simulink model "complete"  (R2019b)
settings: Solver=VariableStepAuto  StartTime=0.0  StopTime=200  RelTol=1e-3
values from neighbouring files (symbols this model uses):
  battery =     [battery.mat]    (also in batteryModel_Sfcn.m = block.DialogPrm(1).Data)
  controllers =     [controllers.mat]
  IC = block.DialogPrm(2).Data    [Dynamics.m]    (also in IC_HoverAt10ftOcto.mat = ; IC_HoverAt10ftOctoWithMotorControl.mat = )
  Motor =     [DJI4114_400kv_BLDC_Motor.mat]
  octomodel =     [octoModel.mat]
undefined symbols (not defined in the file or in its folder): DiscIntNeverNeededParam
libraries: simulink x1
(part 1 of 2)
settings Model: Creator=Researcher  LastModifiedBy=darrahts
settings DataIOCC: ReturnWorkspaceOutputs=off
settings DebuggingCC: ArithmeticOperatorsInVariantConditions=warning
settings SFSimCC: SimUseLocalCustomCode=off  CustomCodeUndefinedFunction=UseInterfaceOnly
settings RTWCC: RTWUseLocalCustomCode=off

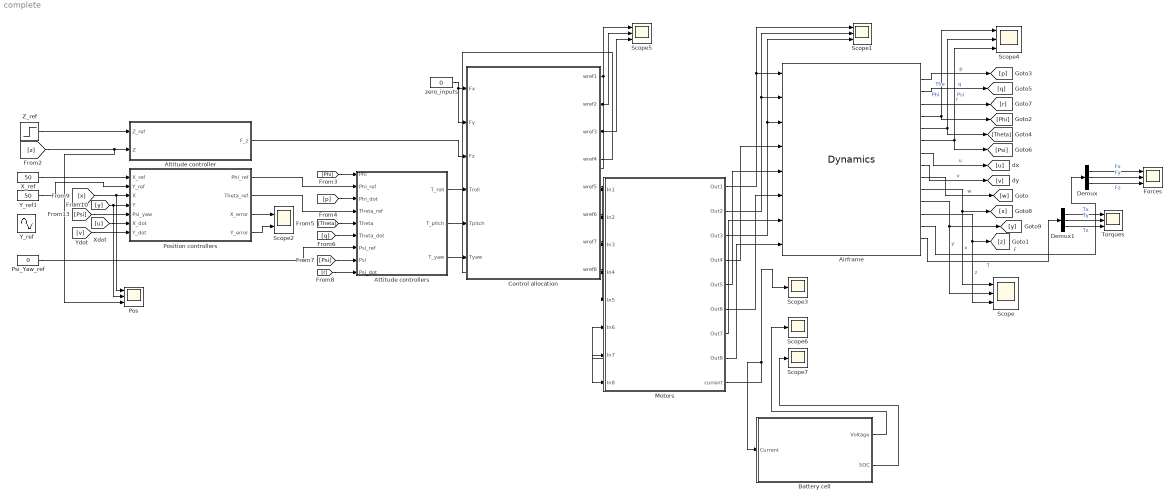
== system complete ==
  Airframe : M-S-Function  FunctionName=Dynamics  Parameters=octomodel, IC
  Altitude controller : Subsystem
  Attitude controllers : Subsystem
  Battery cell : Subsystem
  Control allocation : MATLAB Function  TreatAsAtomicUnit=on
  Demux : Demux  Outputs=3
  Demux1 : Demux  Outputs=3
  Forces : Scope  NumInputPorts=3
  Motors : Subsystem
  Pos : Scope  NumInputPorts=3
  Position controllers : Subsystem
  Psi_Yaw_ref : Constant  Value=0
  Scope{,1,4..5} (4 alike) : Scope  NumInputPorts=3
  Scope2 : Scope  NumInputPorts=2
  Scope3 : Scope
  Scope6 : Scope
  Scope7 : Scope
  Torques : Scope  NumInputPorts=3
  X_ref : Constant  Value=50
  Y_ref : Sin  Amplitude=2  Frequency=0.1  SampleTime=0
  Y_ref1 : Constant  Value=50
  Z_ref : Step  Before=3  After=3  SampleTime=0
  zero_inputs : Constant  Value=0
  wires:
  Airframe/1 -> [p]  "p"
  Airframe/2 -> [q]  "q"
  Airframe/3 -> [r]  "r"
  Airframe/4 -> [Phi], Scope4/1  "Phi"
  Airframe/5 -> [Theta], Scope4/2  "The"
  Airframe/6 -> [Psi], Scope4/3  "Psi"
  Airframe/11 -> [y], Scope/2  "y"
  Airframe/12 -> [z], Scope/3  "z"
  Airframe/7 -> [u]  "u"
  Airframe/10 -> [x], Scope/1  "x"
  Airframe/9 -> [w]  "w"
  Airframe/8 -> [v]  "v"
  Motors/3(Out3) -> Scope1/3, Airframe/3
  Control allocation/1(wref1) -> Scope5/1, Motors/1(In1)
  Control allocation/2(wref2) -> Scope5/2, Motors/2(In2)
  Motors/1(Out1) -> Scope1/1, Airframe/1
  Control allocation/3(wref3) -> Scope5/3, Motors/3(In3)
  Control allocation/4(wref4) -> Motors/4(In4)
  Control allocation/5(wref5) -> Motors/5(In5)
  Control allocation/6(wref6) -> Motors/6(In6)
  Control allocation/7(wref7) -> Motors/7(In7)
  Control allocation/8(wref8) -> Motors/8(In8)
  Motors/8(Out8) -> Airframe/8
  Motors/7(Out7) -> Airframe/7
  Motors/6(Out6) -> Airframe/6
  Motors/5(Out5) -> Airframe/5
  Motors/4(Out4) -> Airframe/4
  Motors/2(Out2) -> Scope1/2, Airframe/2
  zero_inputs/1 -> Control allocation/2(Fy), Control allocation/1(Fx)
  [y] -> Position controllers/4(Y), Pos/2
  Y_ref1/1 -> Position controllers/2(Y_ref)
  X_ref/1 -> Position controllers/1(X_ref)
  [x] -> Pos/1, Position controllers/3(X)
  [Psi] -> Position controllers/5(Psi_yaw)
  [v] -> Position controllers/7(Y_dot)
  [u] -> Position controllers/6(X_dot)
  Position controllers/3(X_error) -> Scope2/1
  Position controllers/4(Y_error) -> Scope2/2
  Z_ref/1 -> Altitude controller/1(Z_ref)
  [z] -> Pos/3, Altitude controller/2(Z)
  Altitude controller/1(F_z) -> Control allocation/3(Fz)
  [Phi] -> Attitude controllers/1(Phi)
  Position controllers/1(Phi_ref) -> Attitude controllers/2(Phi_ref)
  [p] -> Attitude controllers/3(Phi_dot)
  Position controllers/2(Theta_ref) -> Attitude controllers/4(Theta_ref)
  [Theta] -> Attitude controllers/5(Theta)
  [q] -> Attitude controllers/6(Theta_dot)
  Psi_Yaw_ref/1 -> Attitude controllers/7(Psi_ref)
  [Psi] -> Attitude controllers/8(Psi)
  [r] -> Attitude controllers/9(Psi_dot)
  Attitude controllers/1(T_roll) -> Control allocation/4(Troll)
  Attitude controllers/2(T_pitch) -> Control allocation/5(Tpitch)
  Attitude controllers/3(T_yaw) -> Control allocation/6(Tyaw)
  Motors/9(current) -> Scope3/1, Battery cell/1(Current)
  Battery cell/1(Voltage) -> Scope6/1
  Battery cell/2(SOC) -> Scope7/1
  Airframe/13 -> Demux/1  "F"
  Airframe/14 -> Demux1/1  "T"
  Demux/1 -> Forces/1  "Fx"
  Demux/2 -> Forces/2  "Fy"
  Demux/3 -> Forces/3  "Fz"
  Demux1/1 -> Torques/1  "Tx"
  Demux1/2 -> Torques/2  "Ty"
  Demux1/3 -> Torques/3  "Tz"

== system complete/Altitude controller ==
  Z_ref : Inport
  Z : Inport  Port=2
  Add : Sum
  Add2 : Sum  Inputs=+-
  Constant2 : Constant  Value=octomodel.g*octomodel.mass
  PID Controller : simulink/Continuous/PID Controller  Controller=PID  Form=Parallel  TimeDomain=Discrete-time  SampleTime=0.01  IntegratorMethod=Forward Euler  FilterMethod=Forward Euler  ControllerParametersSource=internal  P=controllers.altitude.kp  I=controllers.altitude.ki  D=controllers.altitude.kd  UseFilter=on  N=100  TunerSelectOption=Transfer Function Based (PID Tuner App)  InitialConditionSource=internal  InitialConditionForIntegrator=0  InitialConditionForFilter=0  DifferentiatorICPrevScaledInput=0  ExternalReset=none  TrackingMode=off  Kt=1  LimitOutput=off  UpperSaturationLimit=inf  LowerSaturationLimit=0  LinearizeAsGain=on  AntiWindupMode=none  Kb=1  POutMin=[]  POutMax=[]  IOutMin=[]  IOutMax=[]  DOutMin=[]  DOutMax=[]  NOutMin=[]  NOutMax=[]  SumOutMin=[]  SumOutMax=[]  SaturationOutMin=[]  SaturationOutMax=[]  PParamMin=[]  PParamMax=[]  IParamMin=[]  IParamMax=[]  DParamMin=[]  DParamMax=[]  NParamMin=[]  NParamMax=[]  KbParamMin=[]  KbParamMax=[]  KtParamMin=[]  KtParamMax=[]  KbOutMin=[]  KbOutMax=[]  KtOutMin=[]  KtOutMax=[]  IntegratorOutMin=[]  IntegratorOutMax=[]  FilterOutMin=[]  FilterOutMax=[]  SumI1OutMin=[]  SumI1OutMax=[]  SumI2OutMin=[]  SumI2OutMax=[]  SumI3OutMin=[]  SumI3OutMax=[]  SumI4OutMin=[]  SumI4OutMax=[]  SumDOutMin=[]  SumDOutMax=[]  DifferentiatorOutMin=[]  DifferentiatorOutMax=[]  FilterDiffOutCoefMin=[]  FilterDiffOutCoefMax=[]  ReciprocalOutMin=[]  ReciprocalOutMax=[]  SumDenOutMin=[]  SumDenOutMax=[]  SumNumOutMin=[]  SumNumOutMax=[]  DivideOutMin=[]  DivideOutMax=[]  IntegratorContinuousStateAttributes=''  IntegratorStateMustResolveToSignalObject=off  IntegratorRTWStateStorageClass=Auto  FilterContinuousStateAttributes=''  FilterStateMustResolveToSignalObject=off  FilterRTWStateStorageClass=Auto  ParallelPVariant=InternalParameters  IdealPVariant=Disabled  IVariant=InternalParameters  DVariant=InternalParameters  IntegratorVariant=Discrete  SatVariant=Disabled  AWVariant=Passthrough  PCopyVariant=Disabled  TRVariant=Disabled  FdbkBlocksVariant=Forward  IdealPFdbkVariant=Disabled  SatFdbkVariant=Disabled  DerivativeFilterVariant=ForwardEulerFilter  NVariant=InternalParameters  NCopyVariant=Disabled  FilterICVariant=InternalICsFilter  IntegratorICVariant=InternalICs  ExternalResetVariant=Disabled  TRSumVariant=Passthrough  SumFdbkVariant=Disabled  SumVariant=Sum_PID
  F_z : Outport  VectorParamsAs1DForOutWhenUnconnected=off
  wires:
  Add2/1 -> PID Controller/1
  Constant2/1 -> Add/1
  Z/1 -> Add2/2
  Add/1 -> F_z/1
  Z_ref/1 -> Add2/1
  PID Controller/1 -> Add/2

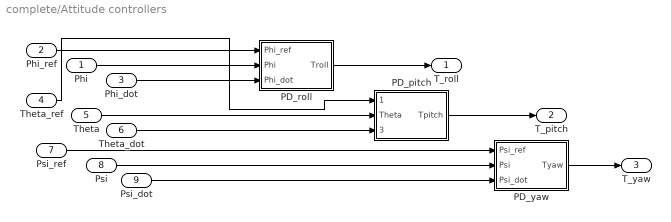
== system complete/Attitude controllers ==
  Phi : Inport
  Phi_ref : Inport  Port=2
  Phi_dot : Inport  Port=3
  Theta_ref : Inport  Port=4
  Theta : Inport  Port=5
  Theta_dot : Inport  Port=6
  Psi_ref : Inport  Port=7
  Psi : Inport  Port=8
  Psi_dot : Inport  Port=9
  PD_pitch : Subsystem
  PD_roll : Subsystem
  PD_yaw : Subsystem
  T_roll : Outport  VectorParamsAs1DForOutWhenUnconnected=off
  T_pitch : Outport  Port=2  VectorParamsAs1DForOutWhenUnconnected=off
  T_yaw : Outport  Port=3  VectorParamsAs1DForOutWhenUnconnected=off
  wires:
  PD_yaw/1(Tyaw) -> T_yaw/1
  PD_roll/1(Troll) -> T_roll/1
  Theta_ref/1 -> PD_pitch/1(Theta_ref)
  Theta_dot/1 -> PD_pitch/3(Theta_dot)
  PD_pitch/1(Tpitch) -> T_pitch/1
  Phi/1 -> PD_roll/2(Phi)
  Psi_dot/1 -> PD_yaw/3(Psi_dot)
  Psi_ref/1 -> PD_yaw/1(Psi_ref)
  Theta/1 -> PD_pitch/2(Theta)
  Phi_dot/1 -> PD_roll/3(Phi_dot)
  Psi/1 -> PD_yaw/2(Psi)
  Phi_ref/1 -> PD_roll/1(Phi_ref)

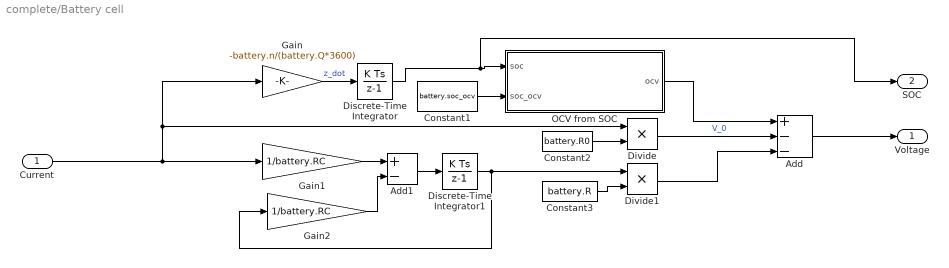
== system complete/Battery cell ==
  Current : Inport
  Add : Sum  Inputs=+--
  Add1 : Sum  Inputs=+-
  Constant1 : Constant  Value=battery.soc_ocv
  Constant2 : Constant  Value=battery.R0
  Constant3 : Constant  Value=battery.R
  Discrete-Time Integrator : DiscreteIntegrator  InitialCondition=1  ICPrevOutput=DiscIntNeverNeededParam  ICPrevScaledInput=DiscIntNeverNeededParam
  Discrete-Time Integrator1 : DiscreteIntegrator  ICPrevOutput=DiscIntNeverNeededParam  ICPrevScaledInput=DiscIntNeverNeededParam
  Divide : Product  Inputs=**
  Divide1 : Product  Inputs=**
  Gain : Gain  Gain=-battery.n/(battery.Q*3600)
  Gain1 : Gain  Gain=1/battery.RC
  Gain2 : Gain  Gain=1/battery.RC
  OCV from SOC : MATLAB Function  TreatAsAtomicUnit=on
  Voltage : Outport  VectorParamsAs1DForOutWhenUnconnected=off
  SOC : Outport  Port=2  VectorParamsAs1DForOutWhenUnconnected=off
  wires:
  Constant2/1 -> Divide/2
  Constant1/1 -> OCV from SOC/2(soc_ocv)
  Divide/1 -> Add/2  "V_0"
  OCV from SOC/1(ocv) -> Add/1
  Add1/1 -> Discrete-Time Integrator1/1
  Gain1/1 -> Add1/1
  Constant3/1 -> Divide1/2
  Divide1/1 -> Add/3
  Gain2/1 -> Add1/2
  Discrete-Time Integrator/1 -> SOC/1, OCV from SOC/1(soc)
  Gain/1 -> Discrete-Time Integrator/1  "z_dot"
  Discrete-Time Integrator1/1 -> Gain2/1, Divide1/1
  Add/1 -> Voltage/1
  Current/1 -> Gain1/1, Gain/1, Divide/1

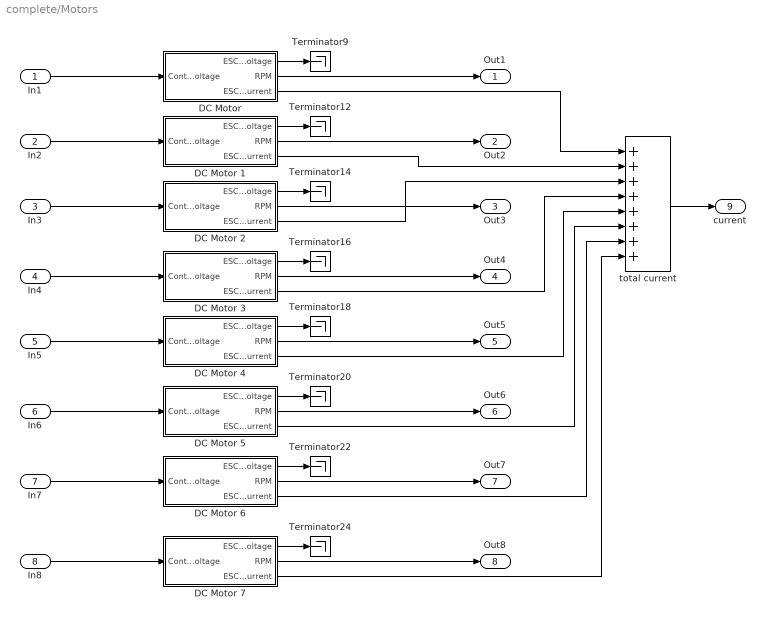
== system complete/Motors ==
  In1 : Inport
  In2 : Inport  Port=2
  In3 : Inport  Port=3
  In4 : Inport  Port=4
  In5 : Inport  Port=5
  In6 : Inport  Port=6
  In7 : Inport  Port=7
  In8 : Inport  Port=8
  "DC Motor " : Subsystem
  DC Motor 1 : Subsystem
  DC Motor 2 : Subsystem
  DC Motor 3 : Subsystem
  DC Motor 4 : Subsystem
  DC Motor 5 : Subsystem
  DC Motor 6 : Subsystem
  DC Motor 7 : Subsystem
  Terminator{9,12,14,16,18,20,22,24} (8 alike) : Terminator
  total current : Sum  Inputs=++++++++
  Out1 : Outport  VectorParamsAs1DForOutWhenUnconnected=off
  Out2 : Outport  Port=2  VectorParamsAs1DForOutWhenUnconnected=off
  Out3 : Outport  Port=3  VectorParamsAs1DForOutWhenUnconnected=off
  Out4 : Outport  Port=4  VectorParamsAs1DForOutWhenUnconnected=off
  Out5 : Outport  Port=5  VectorParamsAs1DForOutWhenUnconnected=off
  Out6 : Outport  Port=6  VectorParamsAs1DForOutWhenUnconnected=off
  Out7 : Outport  Port=7  VectorParamsAs1DForOutWhenUnconnected=off
  Out8 : Outport  Port=8  VectorParamsAs1DForOutWhenUnconnected=off
  current : Outport  Port=9  VectorParamsAs1DForOutWhenUnconnected=off
  wires:
  DC Motor 4/1(ESC Voltage) -> Terminator18/1
  DC Motor 5/3(ESC Current) -> total current/6
  DC Motor 6/3(ESC Current) -> total current/7
  DC Motor 6/1(ESC Voltage) -> Terminator22/1
  DC Motor 5/1(ESC Voltage) -> Terminator20/1
  DC Motor 4/3(ESC Current) -> total current/5
  DC Motor 7/3(ESC Current) -> total current/8
  "DC Motor "/3(ESC Current) -> total current/1
  "DC Motor "/1(ESC Voltage) -> Terminator9/1
  DC Motor 1/3(ESC Current) -> total current/2
  DC Motor 1/1(ESC Voltage) -> Terminator12/1
  DC Motor 2/1(ESC Voltage) -> Terminator14/1
  DC Motor 3/3(ESC Current) -> total current/4
  DC Motor 2/3(ESC Current) -> total current/3
  DC Motor 4/2(RPM) -> Out5/1
  DC Motor 3/1(ESC Voltage) -> Terminator16/1
  DC Motor 7/1(ESC Voltage) -> Terminator24/1
  DC Motor 6/2(RPM) -> Out7/1
  DC Motor 1/2(RPM) -> Out2/1
  DC Motor 2/2(RPM) -> Out3/1
  DC Motor 3/2(RPM) -> Out4/1
  DC Motor 5/2(RPM) -> Out6/1
  DC Motor 7/2(RPM) -> Out8/1
  "DC Motor "/2(RPM) -> Out1/1
  In1/1 -> "DC Motor "/1(Control  Voltage)
  In7/1 -> DC Motor 6/1(Control  Voltage)
  In8/1 -> DC Motor 7/1(Control  Voltage)
  In6/1 -> DC Motor 5/1(Control  Voltage)
  In5/1 -> DC Motor 4/1(Control  Voltage)
  In4/1 -> DC Motor 3/1(Control  Voltage)
  In3/1 -> DC Motor 2/1(Control  Voltage)
  In2/1 -> DC Motor 1/1(Control Voltage)
  total current/1 -> current/1

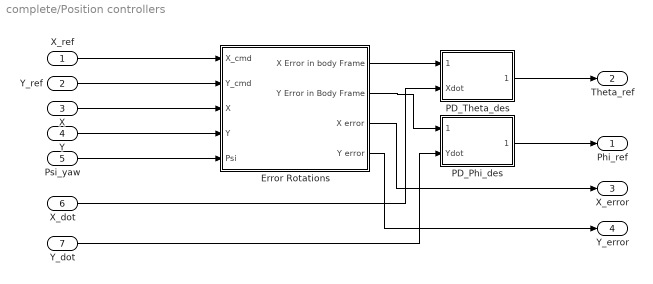
== system complete/Position controllers ==
  X_ref : Inport
  Y_ref : Inport  Port=2
  X : Inport  Port=3
  Y : Inport  Port=4
  Psi_yaw : Inport  Port=5
  X_dot : Inport  Port=6
  Y_dot : Inport  Port=7
  Error Rotations : Subsystem
  PD_Phi_des : Subsystem
  PD_Theta_des : Subsystem
  Phi_ref : Outport  VectorParamsAs1DForOutWhenUnconnected=off
  Theta_ref : Outport  Port=2  VectorParamsAs1DForOutWhenUnconnected=off
  X_error : Outport  Port=3  VectorParamsAs1DForOutWhenUnconnected=off
  Y_error : Outport  Port=4  VectorParamsAs1DForOutWhenUnconnected=off
  wires:
  Y/1 -> Error Rotations/4(Y)
  Y_ref/1 -> Error Rotations/2(Y_cmd)
  Error Rotations/4("Y error ") -> Y_error/1
  Error Rotations/3(X error) -> X_error/1
  Error Rotations/1(X Error in body Frame) -> PD_Theta_des/1(Xdot_ref)
  X/1 -> Error Rotations/3(X)
  Y_dot/1 -> PD_Phi_des/2(Ydot)
  PD_Phi_des/1(Phi_des) -> Phi_ref/1
  Error Rotations/2(Y Error in Body Frame) -> PD_Phi_des/1(Ydot_ref)
  Psi_yaw/1 -> Error Rotations/5(Psi)
  PD_Theta_des/1(Theta_des) -> Theta_ref/1
  X_dot/1 -> PD_Theta_des/2(Xdot)
  X_ref/1 -> Error Rotations/1(X_cmd)

== system complete/Attitude controllers/PD_pitch ==
  Theta_ref : Inport
  Theta : Inport  Port=2
  Theta_dot : Inport  Port=3
  Add : Sum  Inputs=-+
  Gain : Gain  Gain=controllers.attitude.pitch.kp
  Gain1 : Gain  Gain=controllers.attitude.pitch.kp
  Gain2 : Gain  Gain=-1
  Sum : Sum  Inputs=|++
  Tpitch : Outport  VectorParamsAs1DForOutWhenUnconnected=off
  wires:
  Gain2/1 -> Tpitch/1
  Gain/1 -> Sum/1
  Theta/1 -> Add/2
  Add/1 -> Gain/1
  Gain1/1 -> Sum/2
  Sum/1 -> Gain2/1
  Theta_dot/1 -> Gain1/1
  Theta_ref/1 -> Add/1

== system complete/Attitude controllers/PD_roll ==
  Phi_ref : Inport
  Phi : Inport  Port=2
  Phi_dot : Inport  Port=3
  Add : Sum  Inputs=-+
  Gain : Gain  Gain=controllers.attitude.roll.kp
  Gain1 : Gain  Gain=controllers.attitude.roll.kd
  Gain2 : Gain  Gain=-1
  Sum : Sum  Inputs=|++
  Troll : Outport  VectorParamsAs1DForOutWhenUnconnected=off
  wires:
  Phi_ref/1 -> Add/1
  Phi_dot/1 -> Gain1/1
  Sum/1 -> Gain2/1
  Gain1/1 -> Sum/2
  Add/1 -> Gain/1
  Phi/1 -> Add/2
  Gain/1 -> Sum/1
  Gain2/1 -> Troll/1

== system complete/Attitude controllers/PD_yaw ==
  Psi_ref : Inport
  Psi : Inport  Port=2
  Psi_dot : Inport  Port=3
  Add : Sum  Inputs=-+
  Gain : Gain  Gain=controllers.attitude.yaw.kp
  Gain1 : Gain  Gain=controllers.attitude.yaw.kp
  Gain2 : Gain  Gain=-1
  Sum : Sum  Inputs=|++
  Tyaw : Outport  VectorParamsAs1DForOutWhenUnconnected=off
  wires:
  Psi_ref/1 -> Add/1
  Psi_dot/1 -> Gain1/1
  Sum/1 -> Gain2/1
  Gain1/1 -> Sum/2
  Add/1 -> Gain/1
  Psi/1 -> Add/2
  Gain/1 -> Sum/1
  Gain2/1 -> Tyaw/1

== system complete/Motors/DC Motor  ==
  Control  Voltage : Inport
  Convert rad/s to rmp : Gain  Gain=60/(2*pi)
  Electrical part : Subsystem
  Mechanical part : Subsystem
  Scope : Scope
  Scope3 : Scope
  Scope7 : Scope  NumInputPorts=3
  StaticTfric : Constant  Value=0
  ESC Voltage : Outport  VectorParamsAs1DForOutWhenUnconnected=off
  RPM : Outport  Port=2  VectorParamsAs1DForOutWhenUnconnected=off
  ESC Current : Outport  Port=3  VectorParamsAs1DForOutWhenUnconnected=off
  wires:
  StaticTfric/1 -> Mechanical part/1(Static Friction Torque)
  Convert rad/s to rmp/1 -> RPM/1
  Electrical part/1(Electrical Torque) -> Scope3/1, Mechanical part/2(Electrical Torque)
  Mechanical part/1(w angular speed) -> Electrical part/2(w angular speed), Scope7/1, Convert rad/s to rmp/1
  Mechanical part/3(Torque) -> Scope7/3
  Mechanical part/2(Thrust) -> Scope/1, Scope7/2
  Electrical part/2(current) -> ESC Current/1
  Control  Voltage/1 -> ESC Voltage/1, Electrical part/1(ESC voltage)

== system complete/Motors/DC Motor 1 ==
  Control Voltage : Inport
  Convert rad/s to rmp : Gain  Gain=60/(2*pi)
  Electrical part : Subsystem
  Mechanical part : Subsystem
  Scope : Scope
  Scope3 : Scope
  Scope7 : Scope  NumInputPorts=3
  StaticTfric : Constant  Value=0
  ESC Voltage : Outport  VectorParamsAs1DForOutWhenUnconnected=off
  RPM : Outport  Port=2  VectorParamsAs1DForOutWhenUnconnected=off
  ESC Current : Outport  Port=3  VectorParamsAs1DForOutWhenUnconnected=off
  wires:
  Control Voltage/1 -> Electrical part/1(ESC voltage), ESC Voltage/1
  Electrical part/2(current) -> ESC Current/1
  Mechanical part/2(Thrust) -> Scope7/2, Scope/1
  Mechanical part/3(Torque) -> Scope7/3
  Mechanical part/1(w angular speed) -> Convert rad/s to rmp/1, Scope7/1, Electrical part/2(w angular speed)
  Electrical part/1(Electrical Torque) -> Mechanical part/2(Electrical Torque), Scope3/1
  Convert rad/s to rmp/1 -> RPM/1
  StaticTfric/1 -> Mechanical part/1(Static Friction Torque)

== system complete/Motors/DC Motor 2 ==
  Control  Voltage : Inport
  Convert rad/s to rmp : Gain  Gain=60/(2*pi)
  Electrical part : Subsystem
  Mechanical part : Subsystem
  Scope : Scope
  Scope3 : Scope
  Scope7 : Scope  NumInputPorts=3
  StaticTfric : Constant  Value=0
  ESC Voltage : Outport  VectorParamsAs1DForOutWhenUnconnected=off
  RPM : Outport  Port=2  VectorParamsAs1DForOutWhenUnconnected=off
  ESC Current : Outport  Port=3  VectorParamsAs1DForOutWhenUnconnected=off
  wires:
  StaticTfric/1 -> Mechanical part/1(Static Friction Torque)
  Convert rad/s to rmp/1 -> RPM/1
  Electrical part/1(Electrical Torque) -> Scope3/1, Mechanical part/2(Electrical Torque)
  Mechanical part/1(w angular speed) -> Electrical part/2(w angular speed), Scope7/1, Convert rad/s to rmp/1
  Mechanical part/3(Torque) -> Scope7/3
  Mechanical part/2(Thrust) -> Scope/1, Scope7/2
  Electrical part/2(current) -> ESC Current/1
  Control  Voltage/1 -> ESC Voltage/1, Electrical part/1(ESC voltage)

== system complete/Motors/DC Motor 3 ==
  Control  Voltage : Inport
  Convert rad/s to rmp : Gain  Gain=60/(2*pi)
  Electrical part : Subsystem
  Mechanical part : Subsystem
  Scope : Scope
  Scope3 : Scope
  Scope7 : Scope  NumInputPorts=3
  StaticTfric : Constant  Value=0
  ESC Voltage : Outport  VectorParamsAs1DForOutWhenUnconnected=off
  RPM : Outport  Port=2  VectorParamsAs1DForOutWhenUnconnected=off
  ESC Current : Outport  Port=3  VectorParamsAs1DForOutWhenUnconnected=off
  wires:
  Control  Voltage/1 -> Electrical part/1(ESC voltage), ESC Voltage/1
  Electrical part/2(current) -> ESC Current/1
  Mechanical part/2(Thrust) -> Scope7/2, Scope/1
  Mechanical part/3(Torque) -> Scope7/3
  Mechanical part/1(w angular speed) -> Convert rad/s to rmp/1, Scope7/1, Electrical part/2(w angular speed)
  Electrical part/1(Electrical Torque) -> Mechanical part/2(Electrical Torque), Scope3/1
  Convert rad/s to rmp/1 -> RPM/1
  StaticTfric/1 -> Mechanical part/1(Static Friction Torque)

== system complete/Motors/DC Motor 4 ==
  Control  Voltage : Inport
  Convert rad/s to rmp : Gain  Gain=60/(2*pi)
  Electrical part : Subsystem
  Mechanical part : Subsystem
  Scope : Scope
  Scope3 : Scope
  Scope7 : Scope  NumInputPorts=3
  StaticTfric : Constant  Value=0
  ESC Voltage : Outport  VectorParamsAs1DForOutWhenUnconnected=off
  RPM : Outport  Port=2  VectorParamsAs1DForOutWhenUnconnected=off
  ESC Current : Outport  Port=3  VectorParamsAs1DForOutWhenUnconnected=off
  wires:
  StaticTfric/1 -> Mechanical part/1(Static Friction Torque)
  Convert rad/s to rmp/1 -> RPM/1
  Electrical part/1(Electrical Torque) -> Scope3/1, Mechanical part/2(Electrical Torque)
  Mechanical part/1(w angular speed) -> Electrical part/2(w angular speed), Scope7/1, Convert rad/s to rmp/1
  Mechanical part/3(Torque) -> Scope7/3
  Mechanical part/2(Thrust) -> Scope/1, Scope7/2
  Electrical part/2(current) -> ESC Current/1
  Control  Voltage/1 -> ESC Voltage/1, Electrical part/1(ESC voltage)

== system complete/Motors/DC Motor 5 ==
  Control  Voltage : Inport
  Convert rad/s to rmp : Gain  Gain=60/(2*pi)
  Electrical part : Subsystem
  Mechanical part : Subsystem
  Scope : Scope
  Scope3 : Scope
  Scope7 : Scope  NumInputPorts=3
  StaticTfric : Constant  Value=0
  ESC Voltage : Outport  VectorParamsAs1DForOutWhenUnconnected=off
  RPM : Outport  Port=2  VectorParamsAs1DForOutWhenUnconnected=off
  ESC Current : Outport  Port=3  VectorParamsAs1DForOutWhenUnconnected=off
  wires:
  Control  Voltage/1 -> Electrical part/1(ESC voltage), ESC Voltage/1
  Electrical part/2(current) -> ESC Current/1
  Mechanical part/2(Thrust) -> Scope7/2, Scope/1
  Mechanical part/3(Torque) -> Scope7/3
  Mechanical part/1(w angular speed) -> Convert rad/s to rmp/1, Scope7/1, Electrical part/2(w angular speed)
  Electrical part/1(Electrical Torque) -> Mechanical part/2(Electrical Torque), Scope3/1
  Convert rad/s to rmp/1 -> RPM/1
  StaticTfric/1 -> Mechanical part/1(Static Friction Torque)

== system complete/Motors/DC Motor 6 ==
  Control  Voltage : Inport
  Convert rad/s to rmp : Gain  Gain=60/(2*pi)
  Electrical part : Subsystem
  Mechanical part : Subsystem
  Scope : Scope
  Scope3 : Scope
  Scope7 : Scope  NumInputPorts=3
  StaticTfric : Constant  Value=0
  ESC Voltage : Outport  VectorParamsAs1DForOutWhenUnconnected=off
  RPM : Outport  Port=2  VectorParamsAs1DForOutWhenUnconnected=off
  ESC Current : Outport  Port=3  VectorParamsAs1DForOutWhenUnconnected=off
  wires:
  StaticTfric/1 -> Mechanical part/1(Static Friction Torque)
  Convert rad/s to rmp/1 -> RPM/1
  Electrical part/1(Electrical Torque) -> Scope3/1, Mechanical part/2(Electrical Torque)
  Mechanical part/1(w angular speed) -> Electrical part/2(w angular speed), Scope7/1, Convert rad/s to rmp/1
  Mechanical part/3(Torque) -> Scope7/3
  Mechanical part/2(Thrust) -> Scope/1, Scope7/2
  Electrical part/2(current) -> ESC Current/1
  Control  Voltage/1 -> ESC Voltage/1, Electrical part/1(ESC voltage)

== system complete/Motors/DC Motor 7 ==
  Control  Voltage : Inport
  Convert rad/s to rmp : Gain  Gain=60/(2*pi)
  Electrical part : Subsystem
  Mechanical part : Subsystem
  Scope : Scope
  Scope3 : Scope
  Scope7 : Scope  NumInputPorts=3
  StaticTfric : Constant  Value=0
  ESC Voltage : Outport  VectorParamsAs1DForOutWhenUnconnected=off
  RPM : Outport  Port=2  VectorParamsAs1DForOutWhenUnconnected=off
  ESC Current : Outport  Port=3  VectorParamsAs1DForOutWhenUnconnected=off
  wires:
  Control  Voltage/1 -> Electrical part/1(ESC voltage), ESC Voltage/1
  Electrical part/2(current) -> ESC Current/1
  Mechanical part/2(Thrust) -> Scope7/2, Scope/1
  Mechanical part/3(Torque) -> Scope7/3
  Mechanical part/1(w angular speed) -> Convert rad/s to rmp/1, Scope7/1, Electrical part/2(w angular speed)
  Electrical part/1(Electrical Torque) -> Mechanical part/2(Electrical Torque), Scope3/1
  Convert rad/s to rmp/1 -> RPM/1
  StaticTfric/1 -> Mechanical part/1(Static Friction Torque)

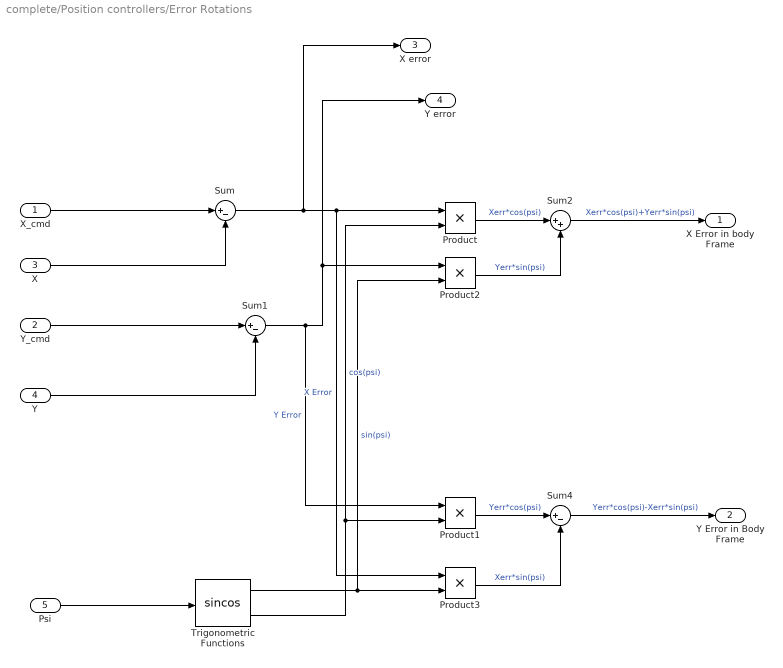
== system complete/Position controllers/Error Rotations ==
  X_cmd : Inport
  Y_cmd : Inport  Port=2
  X : Inport  Port=3
  Y : Inport  Port=4
  Psi : Inport  Port=5
  Product{,1..3} (4 alike) : Product
  Sum : Sum  Inputs=|+-
  Sum1 : Sum  Inputs=|+-
  Sum2 : Sum  Inputs=|++
  Sum4 : Sum  Inputs=|+-
  Trigonometric Functions : Trigonometry  Operator=sincos
  X Error in body Frame : Outport  VectorParamsAs1DForOutWhenUnconnected=off
  Y Error in Body Frame : Outport  Port=2  VectorParamsAs1DForOutWhenUnconnected=off
  X error : Outport  Port=3  VectorParamsAs1DForOutWhenUnconnected=off
  "Y error " : Outport  Port=4  VectorParamsAs1DForOutWhenUnconnected=off
  wires:
  Sum4/1 -> Y Error in Body Frame/1  "Yerr*cos(psi)-Xerr*sin(psi)"
  Product3/1 -> Sum4/2  "Xerr*sin(psi)"
  Sum1/1 -> "Y error "/1, Product2/1, Product1/1  "Y Error"
  Trigonometric Functions/1 -> Product2/2, Product3/2  "sin(psi)"
  Sum2/1 -> X Error in body Frame/1  "Xerr*cos(psi)+Yerr*sin(psi)"
  Y_cmd/1 -> Sum1/1
  X_cmd/1 -> Sum/1
  X/1 -> Sum/2
  Y/1 -> Sum1/2
  Sum/1 -> X error/1, Product3/1, Product/1  "X Error"
  Trigonometric Functions/2 -> Product/2, Product1/2  "cos(psi)"
  Product/1 -> Sum2/1  "Xerr*cos(psi)"
  Product2/1 -> Sum2/2  "Yerr*sin(psi)"
  Product1/1 -> Sum4/1  "Yerr*cos(psi)"
  Psi/1 -> Trigonometric Functions/1

== system complete/Position controllers/PD_Phi_des ==
  Ydot_ref : Inport
  Ydot : Inport  Port=2
  Add : Sum  Inputs=+-
  Gain : Gain
  Gain1 : Gain  Gain=.5
  Gain2 : Gain  Gain=-1
  Saturation in radians : Saturate  UpperLimit=12*pi/180  LowerLimit=-12*pi/180
  Sum : Sum  Inputs=|+-
  Phi_des : Outport  VectorParamsAs1DForOutWhenUnconnected=off
  wires:
  Saturation in radians/1 -> Phi_des/1
  Ydot_ref/1 -> Add/1
  Ydot/1 -> Add/2, Gain1/1
  Gain1/1 -> Sum/2
  Add/1 -> Gain/1
  Gain/1 -> Sum/1
  Sum/1 -> Gain2/1
  Gain2/1 -> Saturation in radians/1

== system complete/Position controllers/PD_Theta_des ==
  Xdot_ref : Inport
  Xdot : Inport  Port=2
  Add : Sum  Inputs=+-
  Gain : Gain
  Gain1 : Gain  Gain=.5
  Saturation in radians : Saturate  UpperLimit=12*pi/180  LowerLimit=-12*pi/180
  Sum : Sum  Inputs=|+-
  Theta_des : Outport  VectorParamsAs1DForOutWhenUnconnected=off
  wires:
  Sum/1 -> Saturation in radians/1
  Gain/1 -> Sum/1
  Add/1 -> Gain/1
  Gain1/1 -> Sum/2
  Xdot/1 -> Gain1/1, Add/2
  Xdot_ref/1 -> Add/1
  Saturation in radians/1 -> Theta_des/1

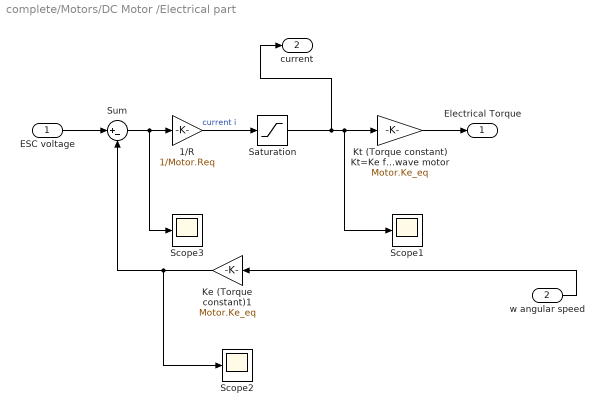
== system complete/Motors/DC Motor /Electrical part ==
  ESC voltage : Inport
  w angular speed : Inport  Port=2
  1/R : Gain  Gain=1/Motor.Req
  Ke (Torque constant)1 : Gain  Gain=Motor.Ke_eq
  Kt (Torque constant) Kt=Ke for an ideal square wave motor : Gain  Gain=Motor.Ke_eq
  Saturation : Saturate  UpperLimit=22  LowerLimit=0
  Scope1 : Scope
  Scope2 : Scope
  Scope3 : Scope
  Sum : Sum  Inputs=|+-
  Electrical Torque : Outport  VectorParamsAs1DForOutWhenUnconnected=off
  current : Outport  Port=2  VectorParamsAs1DForOutWhenUnconnected=off
  wires:
  1/R/1 -> Saturation/1  "current i"
  Sum/1 -> Scope3/1, 1/R/1
  Kt (Torque constant) Kt=Ke for an ideal square wave motor/1 -> Electrical Torque/1
  Ke (Torque constant)1/1 -> Scope2/1, Sum/2
  ESC voltage/1 -> Sum/1
  w angular speed/1 -> Ke (Torque constant)1/1
  Saturation/1 -> Scope1/1, Kt (Torque constant) Kt=Ke for an ideal square wave motor/1, current/1

== system complete/Motors/DC Motor /Mechanical part ==
  Static Friction Torque : Inport
  Electrical Torque : Inport  Port=2
  1/J Inertia constant : Gain  Gain=1/Motor.J
  "Df viscous damping coefficient Dynamic Friction coefficient " : Gain  Gain=Motor.Df
  Discrete-Time Integrator : DiscreteIntegrator  gainval=1  InitialCondition=IC.w1  SampleTime=octomodel.sampletime  ICPrevOutput=DiscIntNeverNeededParam  ICPrevScaledInput=DiscIntNeverNeededParam
  Sum1 : Sum  Inputs=--+-
  speed - torque load relationship we will not consider for now : Subsystem
  w angular speed : Outport  VectorParamsAs1DForOutWhenUnconnected=off
  Thrust : Outport  Port=2  VectorParamsAs1DForOutWhenUnconnected=off
  Torque : Outport  Port=3  VectorParamsAs1DForOutWhenUnconnected=off
  wires:
  1/J Inertia constant/1 -> Discrete-Time Integrator/1
  Static Friction Torque/1 -> Sum1/2
  "Df viscous damping coefficient Dynamic Friction coefficient "/1 -> Sum1/4
  Discrete-Time Integrator/1 -> speed - torque load relationship we will not consider for now/1(w angular speed), w angular speed/1, "Df viscous damping coefficient Dynamic Friction coefficient "/1  "w angular speed"
  Sum1/1 -> 1/J Inertia constant/1
  Electrical Torque/1 -> Sum1/3
  speed - torque load relationship we will not consider for now/2(thrusth) -> Thrust/1
  speed - torque load relationship we will not consider for now/1(torque) -> Sum1/1, Torque/1

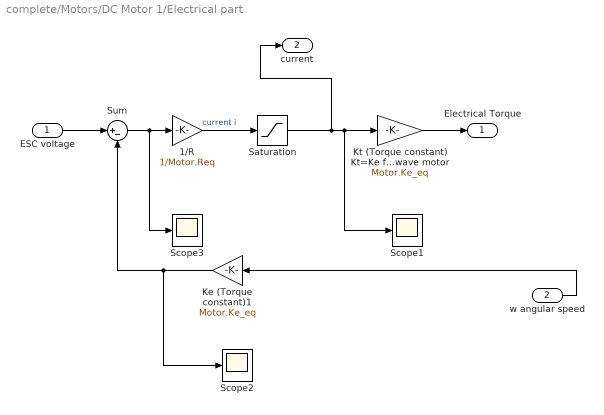
== system complete/Motors/DC Motor 1/Electrical part ==
  ESC voltage : Inport
  w angular speed : Inport  Port=2
  1/R : Gain  Gain=1/Motor.Req
  Ke (Torque constant)1 : Gain  Gain=Motor.Ke_eq
  Kt (Torque constant) Kt=Ke for an ideal square wave motor : Gain  Gain=Motor.Ke_eq
  Saturation : Saturate  UpperLimit=22  LowerLimit=0
  Scope1 : Scope
  Scope2 : Scope
  Scope3 : Scope
  Sum : Sum  Inputs=|+-
  Electrical Torque : Outport  VectorParamsAs1DForOutWhenUnconnected=off
  current : Outport  Port=2  VectorParamsAs1DForOutWhenUnconnected=off
  wires:
  Saturation/1 -> current/1, Kt (Torque constant) Kt=Ke for an ideal square wave motor/1, Scope1/1
  w angular speed/1 -> Ke (Torque constant)1/1
  ESC voltage/1 -> Sum/1
  Ke (Torque constant)1/1 -> Sum/2, Scope2/1
  Kt (Torque constant) Kt=Ke for an ideal square wave motor/1 -> Electrical Torque/1
  Sum/1 -> 1/R/1, Scope3/1
  1/R/1 -> Saturation/1  "current i"

== system complete/Motors/DC Motor 1/Mechanical part ==
  Static Friction Torque : Inport
  Electrical Torque : Inport  Port=2
  1/J Inertia constant : Gain  Gain=1/Motor.J
  "Df viscous damping coefficient Dynamic Friction coefficient " : Gain  Gain=Motor.Df
  Discrete-Time Integrator : DiscreteIntegrator  gainval=1  InitialCondition=IC.w2  SampleTime=octomodel.sampletime  ICPrevOutput=DiscIntNeverNeededParam  ICPrevScaledInput=DiscIntNeverNeededParam
  Sum1 : Sum  Inputs=--+-
  speed - torque load relationship we will not consider for now : Subsystem
  w angular speed : Outport  VectorParamsAs1DForOutWhenUnconnected=off
  Thrust : Outport  Port=2  VectorParamsAs1DForOutWhenUnconnected=off
  Torque : Outport  Port=3  VectorParamsAs1DForOutWhenUnconnected=off
  wires:
  speed - torque load relationship we will not consider for now/1(torque) -> Torque/1, Sum1/1
  speed - torque load relationship we will not consider for now/2(thrusth) -> Thrust/1
  Electrical Torque/1 -> Sum1/3
  Sum1/1 -> 1/J Inertia constant/1
  Discrete-Time Integrator/1 -> "Df viscous damping coefficient Dynamic Friction coefficient "/1, w angular speed/1, speed - torque load relationship we will not consider for now/1(w angular speed)  "w angular speed"
  "Df viscous damping coefficient Dynamic Friction coefficient "/1 -> Sum1/4
  Static Friction Torque/1 -> Sum1/2
  1/J Inertia constant/1 -> Discrete-Time Integrator/1

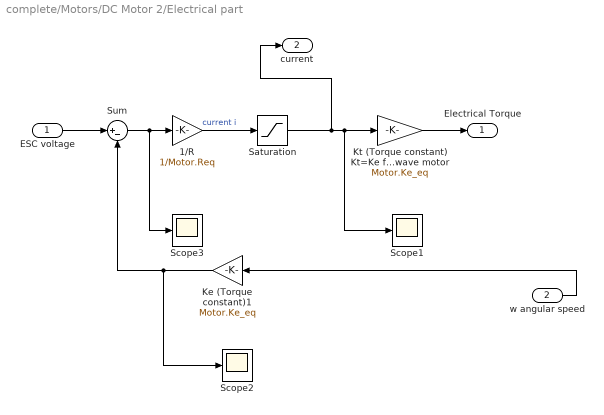
== system complete/Motors/DC Motor 2/Electrical part ==
  ESC voltage : Inport
  w angular speed : Inport  Port=2
  1/R : Gain  Gain=1/Motor.Req
  Ke (Torque constant)1 : Gain  Gain=Motor.Ke_eq
  Kt (Torque constant) Kt=Ke for an ideal square wave motor : Gain  Gain=Motor.Ke_eq
  Saturation : Saturate  UpperLimit=22  LowerLimit=0
  Scope1 : Scope
  Scope2 : Scope
  Scope3 : Scope
  Sum : Sum  Inputs=|+-
  Electrical Torque : Outport  VectorParamsAs1DForOutWhenUnconnected=off
  current : Outport  Port=2  VectorParamsAs1DForOutWhenUnconnected=off
  wires:
  1/R/1 -> Saturation/1  "current i"
  Sum/1 -> Scope3/1, 1/R/1
  Kt (Torque constant) Kt=Ke for an ideal square wave motor/1 -> Electrical Torque/1
  Ke (Torque constant)1/1 -> Scope2/1, Sum/2
  ESC voltage/1 -> Sum/1
  w angular speed/1 -> Ke (Torque constant)1/1
  Saturation/1 -> Scope1/1, Kt (Torque constant) Kt=Ke for an ideal square wave motor/1, current/1

== system complete/Motors/DC Motor 2/Mechanical part ==
  Static Friction Torque : Inport
  Electrical Torque : Inport  Port=2
  1/J Inertia constant : Gain  Gain=1/Motor.J
  "Df viscous damping coefficient Dynamic Friction coefficient " : Gain  Gain=Motor.Df
  Discrete-Time Integrator : DiscreteIntegrator  gainval=1  InitialCondition=IC.w3  SampleTime=octomodel.sampletime  ICPrevOutput=DiscIntNeverNeededParam  ICPrevScaledInput=DiscIntNeverNeededParam
  Sum1 : Sum  Inputs=--+-
  speed - torque load relationship we will not consider for now : Subsystem
  w angular speed : Outport  VectorParamsAs1DForOutWhenUnconnected=off
  Thrust : Outport  Port=2  VectorParamsAs1DForOutWhenUnconnected=off
  Torque : Outport  Port=3  VectorParamsAs1DForOutWhenUnconnected=off
  wires:
  1/J Inertia constant/1 -> Discrete-Time Integrator/1
  Static Friction Torque/1 -> Sum1/2
  "Df viscous damping coefficient Dynamic Friction coefficient "/1 -> Sum1/4
  Discrete-Time Integrator/1 -> speed - torque load relationship we will not consider for now/1(w angular speed), w angular speed/1, "Df viscous damping coefficient Dynamic Friction coefficient "/1  "w angular speed"
  Sum1/1 -> 1/J Inertia constant/1
  Electrical Torque/1 -> Sum1/3
  speed - torque load relationship we will not consider for now/2(thrusth) -> Thrust/1
  speed - torque load relationship we will not consider for now/1(torque) -> Sum1/1, Torque/1

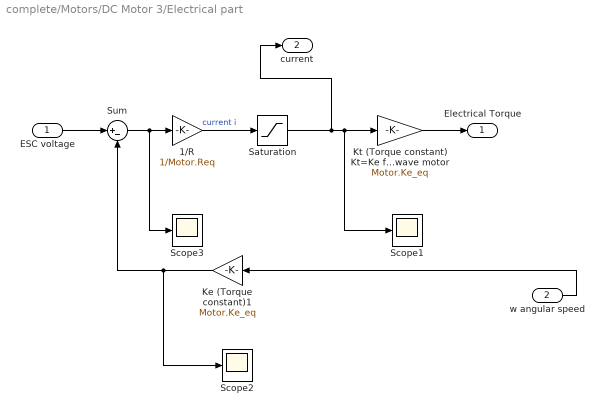
== system complete/Motors/DC Motor 3/Electrical part ==
  ESC voltage : Inport
  w angular speed : Inport  Port=2
  1/R : Gain  Gain=1/Motor.Req
  Ke (Torque constant)1 : Gain  Gain=Motor.Ke_eq
  Kt (Torque constant) Kt=Ke for an ideal square wave motor : Gain  Gain=Motor.Ke_eq
  Saturation : Saturate  UpperLimit=22  LowerLimit=0
  Scope1 : Scope
  Scope2 : Scope
  Scope3 : Scope
  Sum : Sum  Inputs=|+-
  Electrical Torque : Outport  VectorParamsAs1DForOutWhenUnconnected=off
  current : Outport  Port=2  VectorParamsAs1DForOutWhenUnconnected=off
  wires:
  Saturation/1 -> current/1, Kt (Torque constant) Kt=Ke for an ideal square wave motor/1, Scope1/1
  w angular speed/1 -> Ke (Torque constant)1/1
  ESC voltage/1 -> Sum/1
  Ke (Torque constant)1/1 -> Sum/2, Scope2/1
  Kt (Torque constant) Kt=Ke for an ideal square wave motor/1 -> Electrical Torque/1
  Sum/1 -> 1/R/1, Scope3/1
  1/R/1 -> Saturation/1  "current i"

== system complete/Motors/DC Motor 3/Mechanical part ==
  Static Friction Torque : Inport
  Electrical Torque : Inport  Port=2
  1/J Inertia constant : Gain  Gain=1/Motor.J
  "Df viscous damping coefficient Dynamic Friction coefficient " : Gain  Gain=Motor.Df
  Discrete-Time Integrator : DiscreteIntegrator  gainval=1  InitialCondition=IC.w4  SampleTime=octomodel.sampletime  ICPrevOutput=DiscIntNeverNeededParam  ICPrevScaledInput=DiscIntNeverNeededParam
  Sum1 : Sum  Inputs=--+-
  speed - torque load relationship we will not consider for now : Subsystem
  w angular speed : Outport  VectorParamsAs1DForOutWhenUnconnected=off
  Thrust : Outport  Port=2  VectorParamsAs1DForOutWhenUnconnected=off
  Torque : Outport  Port=3  VectorParamsAs1DForOutWhenUnconnected=off
  wires:
  speed - torque load relationship we will not consider for now/1(torque) -> Torque/1, Sum1/1
  speed - torque load relationship we will not consider for now/2(thrusth) -> Thrust/1
  Electrical Torque/1 -> Sum1/3
  Sum1/1 -> 1/J Inertia constant/1
  Discrete-Time Integrator/1 -> "Df viscous damping coefficient Dynamic Friction coefficient "/1, w angular speed/1, speed - torque load relationship we will not consider for now/1(w angular speed)  "w angular speed"
  "Df viscous damping coefficient Dynamic Friction coefficient "/1 -> Sum1/4
  Static Friction Torque/1 -> Sum1/2
  1/J Inertia constant/1 -> Discrete-Time Integrator/1

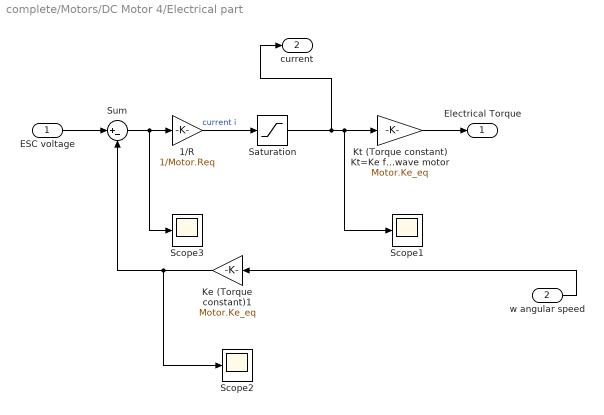
== system complete/Motors/DC Motor 4/Electrical part ==
  ESC voltage : Inport
  w angular speed : Inport  Port=2
  1/R : Gain  Gain=1/Motor.Req
  Ke (Torque constant)1 : Gain  Gain=Motor.Ke_eq
  Kt (Torque constant) Kt=Ke for an ideal square wave motor : Gain  Gain=Motor.Ke_eq
  Saturation : Saturate  UpperLimit=22  LowerLimit=0
  Scope1 : Scope
  Scope2 : Scope
  Scope3 : Scope
  Sum : Sum  Inputs=|+-
  Electrical Torque : Outport  VectorParamsAs1DForOutWhenUnconnected=off
  current : Outport  Port=2  VectorParamsAs1DForOutWhenUnconnected=off
  wires:
  1/R/1 -> Saturation/1  "current i"
  Sum/1 -> Scope3/1, 1/R/1
  Kt (Torque constant) Kt=Ke for an ideal square wave motor/1 -> Electrical Torque/1
  Ke (Torque constant)1/1 -> Scope2/1, Sum/2
  ESC voltage/1 -> Sum/1
  w angular speed/1 -> Ke (Torque constant)1/1
  Saturation/1 -> Scope1/1, Kt (Torque constant) Kt=Ke for an ideal square wave motor/1, current/1

== system complete/Motors/DC Motor 4/Mechanical part ==
  Static Friction Torque : Inport
  Electrical Torque : Inport  Port=2
  1/J Inertia constant : Gain  Gain=1/Motor.J
  "Df viscous damping coefficient Dynamic Friction coefficient " : Gain  Gain=Motor.Df
  Discrete-Time Integrator : DiscreteIntegrator  gainval=1  InitialCondition=IC.w5  SampleTime=octomodel.sampletime  ICPrevOutput=DiscIntNeverNeededParam  ICPrevScaledInput=DiscIntNeverNeededParam
  Sum1 : Sum  Inputs=--+-
  speed - torque load relationship we will not consider for now : Subsystem
  w angular speed : Outport  VectorParamsAs1DForOutWhenUnconnected=off
  Thrust : Outport  Port=2  VectorParamsAs1DForOutWhenUnconnected=off
  Torque : Outport  Port=3  VectorParamsAs1DForOutWhenUnconnected=off
  wires:
  1/J Inertia constant/1 -> Discrete-Time Integrator/1
  Static Friction Torque/1 -> Sum1/2
  "Df viscous damping coefficient Dynamic Friction coefficient "/1 -> Sum1/4
  Discrete-Time Integrator/1 -> speed - torque load relationship we will not consider for now/1(w angular speed), w angular speed/1, "Df viscous damping coefficient Dynamic Friction coefficient "/1  "w angular speed"
  Sum1/1 -> 1/J Inertia constant/1
  Electrical Torque/1 -> Sum1/3
  speed - torque load relationship we will not consider for now/2(thrusth) -> Thrust/1
  speed - torque load relationship we will not consider for now/1(torque) -> Sum1/1, Torque/1

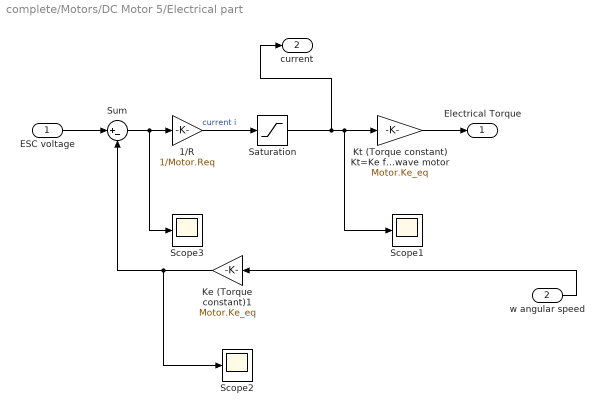
== system complete/Motors/DC Motor 5/Electrical part ==
  ESC voltage : Inport
  w angular speed : Inport  Port=2
  1/R : Gain  Gain=1/Motor.Req
  Ke (Torque constant)1 : Gain  Gain=Motor.Ke_eq
  Kt (Torque constant) Kt=Ke for an ideal square wave motor : Gain  Gain=Motor.Ke_eq
  Saturation : Saturate  UpperLimit=22  LowerLimit=0
  Scope1 : Scope
  Scope2 : Scope
  Scope3 : Scope
  Sum : Sum  Inputs=|+-
  Electrical Torque : Outport  VectorParamsAs1DForOutWhenUnconnected=off
  current : Outport  Port=2  VectorParamsAs1DForOutWhenUnconnected=off
  wires:
  Saturation/1 -> current/1, Kt (Torque constant) Kt=Ke for an ideal square wave motor/1, Scope1/1
  w angular speed/1 -> Ke (Torque constant)1/1
  ESC voltage/1 -> Sum/1
  Ke (Torque constant)1/1 -> Sum/2, Scope2/1
  Kt (Torque constant) Kt=Ke for an ideal square wave motor/1 -> Electrical Torque/1
  Sum/1 -> 1/R/1, Scope3/1
  1/R/1 -> Saturation/1  "current i"

== system complete/Motors/DC Motor 5/Mechanical part ==
  Static Friction Torque : Inport
  Electrical Torque : Inport  Port=2
  1/J Inertia constant : Gain  Gain=1/Motor.J
  "Df viscous damping coefficient Dynamic Friction coefficient " : Gain  Gain=Motor.Df
  Discrete-Time Integrator : DiscreteIntegrator  gainval=1  InitialCondition=IC.w6  SampleTime=octomodel.sampletime  ICPrevOutput=DiscIntNeverNeededParam  ICPrevScaledInput=DiscIntNeverNeededParam
  Sum1 : Sum  Inputs=--+-
  speed - torque load relationship we will not consider for now : Subsystem
  w angular speed : Outport  VectorParamsAs1DForOutWhenUnconnected=off
  Thrust : Outport  Port=2  VectorParamsAs1DForOutWhenUnconnected=off
  Torque : Outport  Port=3  VectorParamsAs1DForOutWhenUnconnected=off
  wires:
  speed - torque load relationship we will not consider for now/1(torque) -> Torque/1, Sum1/1
  speed - torque load relationship we will not consider for now/2(thrusth) -> Thrust/1
  Electrical Torque/1 -> Sum1/3
  Sum1/1 -> 1/J Inertia constant/1
  Discrete-Time Integrator/1 -> "Df viscous damping coefficient Dynamic Friction coefficient "/1, w angular speed/1, speed - torque load relationship we will not consider for now/1(w angular speed)  "w angular speed"
  "Df viscous damping coefficient Dynamic Friction coefficient "/1 -> Sum1/4
  Static Friction Torque/1 -> Sum1/2
  1/J Inertia constant/1 -> Discrete-Time Integrator/1

== system complete/Motors/DC Motor 6/Electrical part ==
  ESC voltage : Inport
  w angular speed : Inport  Port=2
  1/R : Gain  Gain=1/Motor.Req
  Ke (Torque constant)1 : Gain  Gain=Motor.Ke_eq
  Kt (Torque constant) Kt=Ke for an ideal square wave motor : Gain  Gain=Motor.Ke_eq
  Saturation : Saturate  UpperLimit=22  LowerLimit=0
  Scope1 : Scope
  Scope2 : Scope
  Scope3 : Scope
  Sum : Sum  Inputs=|+-
  Electrical Torque : Outport  VectorParamsAs1DForOutWhenUnconnected=off
  current : Outport  Port=2  VectorParamsAs1DForOutWhenUnconnected=off
  wires:
  1/R/1 -> Saturation/1  "current i"
  Sum/1 -> Scope3/1, 1/R/1
  Kt (Torque constant) Kt=Ke for an ideal square wave motor/1 -> Electrical Torque/1
  Ke (Torque constant)1/1 -> Scope2/1, Sum/2
  ESC voltage/1 -> Sum/1
  w angular speed/1 -> Ke (Torque constant)1/1
  Saturation/1 -> Scope1/1, Kt (Torque constant) Kt=Ke for an ideal square wave motor/1, current/1

== system complete/Motors/DC Motor 6/Mechanical part ==
  Static Friction Torque : Inport
  Electrical Torque : Inport  Port=2
  1/J Inertia constant : Gain  Gain=1/Motor.J
  "Df viscous damping coefficient Dynamic Friction coefficient " : Gain  Gain=Motor.Df
  Discrete-Time Integrator : DiscreteIntegrator  gainval=1  InitialCondition=IC.w7  SampleTime=octomodel.sampletime  ICPrevOutput=DiscIntNeverNeededParam  ICPrevScaledInput=DiscIntNeverNeededParam
  Sum1 : Sum  Inputs=--+-
  speed - torque load relationship we will not consider for now : Subsystem
  w angular speed : Outport  VectorParamsAs1DForOutWhenUnconnected=off
  Thrust : Outport  Port=2  VectorParamsAs1DForOutWhenUnconnected=off
  Torque : Outport  Port=3  VectorParamsAs1DForOutWhenUnconnected=off
  wires:
  1/J Inertia constant/1 -> Discrete-Time Integrator/1
  Static Friction Torque/1 -> Sum1/2
  "Df viscous damping coefficient Dynamic Friction coefficient "/1 -> Sum1/4
  Discrete-Time Integrator/1 -> speed - torque load relationship we will not consider for now/1(w angular speed), w angular speed/1, "Df viscous damping coefficient Dynamic Friction coefficient "/1  "w angular speed"
  Sum1/1 -> 1/J Inertia constant/1
  Electrical Torque/1 -> Sum1/3
  speed - torque load relationship we will not consider for now/2(thrusth) -> Thrust/1
  speed - torque load relationship we will not consider for now/1(torque) -> Sum1/1, Torque/1

== system complete/Motors/DC Motor 7/Electrical part ==
  ESC voltage : Inport
  w angular speed : Inport  Port=2
  1/R : Gain  Gain=1/Motor.Req
  Ke (Torque constant)1 : Gain  Gain=Motor.Ke_eq
  Kt (Torque constant) Kt=Ke for an ideal square wave motor : Gain  Gain=Motor.Ke_eq
  Saturation : Saturate  UpperLimit=22  LowerLimit=0
  Scope1 : Scope
  Scope2 : Scope
  Scope3 : Scope
  Sum : Sum  Inputs=|+-
  Electrical Torque : Outport  VectorParamsAs1DForOutWhenUnconnected=off
  current : Outport  Port=2  VectorParamsAs1DForOutWhenUnconnected=off
  wires:
  Saturation/1 -> current/1, Kt (Torque constant) Kt=Ke for an ideal square wave motor/1, Scope1/1
  w angular speed/1 -> Ke (Torque constant)1/1
  ESC voltage/1 -> Sum/1
  Ke (Torque constant)1/1 -> Sum/2, Scope2/1
  Kt (Torque constant) Kt=Ke for an ideal square wave motor/1 -> Electrical Torque/1
  Sum/1 -> 1/R/1, Scope3/1
  1/R/1 -> Saturation/1  "current i"

== system complete/Motors/DC Motor 7/Mechanical part ==
  Static Friction Torque : Inport
  Electrical Torque : Inport  Port=2
  1/J Inertia constant : Gain  Gain=1/Motor.J
  "Df viscous damping coefficient Dynamic Friction coefficient " : Gain  Gain=Motor.Df
  Discrete-Time Integrator : DiscreteIntegrator  gainval=1  InitialCondition=IC.w8  SampleTime=octomodel.sampletime  ICPrevOutput=DiscIntNeverNeededParam  ICPrevScaledInput=DiscIntNeverNeededParam
  Sum1 : Sum  Inputs=--+-
  speed - torque load relationship we will not consider for now : Subsystem
  w angular speed : Outport  VectorParamsAs1DForOutWhenUnconnected=off
  Thrust : Outport  Port=2  VectorParamsAs1DForOutWhenUnconnected=off
  Torque : Outport  Port=3  VectorParamsAs1DForOutWhenUnconnected=off
  wires:
  speed - torque load relationship we will not consider for now/1(torque) -> Torque/1, Sum1/1
  speed - torque load relationship we will not consider for now/2(thrusth) -> Thrust/1
  Electrical Torque/1 -> Sum1/3
  Sum1/1 -> 1/J Inertia constant/1
  Discrete-Time Integrator/1 -> "Df viscous damping coefficient Dynamic Friction coefficient "/1, w angular speed/1, speed - torque load relationship we will not consider for now/1(w angular speed)  "w angular speed"
  "Df viscous damping coefficient Dynamic Friction coefficient "/1 -> Sum1/4
  Static Friction Torque/1 -> Sum1/2
  1/J Inertia constant/1 -> Discrete-Time Integrator/1

== system complete/Motors/DC Motor /Mechanical part/speed - torque load relationship we will not consider for now ==
  w angular speed : Inport
  Convert rad/s to rmp : Gain  Gain=60/(2*pi)
  "Propeller model " : MATLAB Function  TreatAsAtomicUnit=on  SystemSampleTime=octomodel.sampletime
  torque : Outport  VectorParamsAs1DForOutWhenUnconnected=off
  thrusth : Outport  Port=2  VectorParamsAs1DForOutWhenUnconnected=off
  wires:
  Convert rad/s to rmp/1 -> "Propeller model "/1(rpm)
  w angular speed/1 -> Convert rad/s to rmp/1
  "Propeller model "/2(thrust) -> thrusth/1
  "Propeller model "/1(torque) -> torque/1

== system complete/Motors/DC Motor 1/Mechanical part/speed - torque load relationship we will not consider for now ==
  w angular speed : Inport
  Convert rad/s to rmp : Gain  Gain=60/(2*pi)
  "Propeller model " : MATLAB Function  TreatAsAtomicUnit=on  SystemSampleTime=octomodel.sampletime
  torque : Outport  VectorParamsAs1DForOutWhenUnconnected=off
  thrusth : Outport  Port=2  VectorParamsAs1DForOutWhenUnconnected=off
  wires:
  "Propeller model "/1(torque) -> torque/1
  "Propeller model "/2(thrust) -> thrusth/1
  w angular speed/1 -> Convert rad/s to rmp/1
  Convert rad/s to rmp/1 -> "Propeller model "/1(rpm)

== system complete/Motors/DC Motor 2/Mechanical part/speed - torque load relationship we will not consider for now ==
  w angular speed : Inport
  Convert rad/s to rmp : Gain  Gain=60/(2*pi)
  "Propeller model " : MATLAB Function  TreatAsAtomicUnit=on  SystemSampleTime=octomodel.sampletime
  torque : Outport  VectorParamsAs1DForOutWhenUnconnected=off
  thrusth : Outport  Port=2  VectorParamsAs1DForOutWhenUnconnected=off
  wires:
  Convert rad/s to rmp/1 -> "Propeller model "/1(rpm)
  w angular speed/1 -> Convert rad/s to rmp/1
  "Propeller model "/2(thrust) -> thrusth/1
  "Propeller model "/1(torque) -> torque/1

== system complete/Motors/DC Motor 3/Mechanical part/speed - torque load relationship we will not consider for now ==
  w angular speed : Inport
  Convert rad/s to rmp : Gain  Gain=60/(2*pi)
  "Propeller model " : MATLAB Function  TreatAsAtomicUnit=on  SystemSampleTime=octomodel.sampletime
  torque : Outport  VectorParamsAs1DForOutWhenUnconnected=off
  thrusth : Outport  Port=2  VectorParamsAs1DForOutWhenUnconnected=off
  wires:
  "Propeller model "/1(torque) -> torque/1
  "Propeller model "/2(thrust) -> thrusth/1
  w angular speed/1 -> Convert rad/s to rmp/1
  Convert rad/s to rmp/1 -> "Propeller model "/1(rpm)

== system complete/Motors/DC Motor 4/Mechanical part/speed - torque load relationship we will not consider for now ==
  w angular speed : Inport
  Convert rad/s to rmp : Gain  Gain=60/(2*pi)
  "Propeller model " : MATLAB Function  TreatAsAtomicUnit=on  SystemSampleTime=octomodel.sampletime
  torque : Outport  VectorParamsAs1DForOutWhenUnconnected=off
  thrusth : Outport  Port=2  VectorParamsAs1DForOutWhenUnconnected=off
  wires:
  Convert rad/s to rmp/1 -> "Propeller model "/1(rpm)
  w angular speed/1 -> Convert rad/s to rmp/1
  "Propeller model "/2(thrust) -> thrusth/1
  "Propeller model "/1(torque) -> torque/1

== system complete/Motors/DC Motor 5/Mechanical part/speed - torque load relationship we will not consider for now ==
  w angular speed : Inport
  Convert rad/s to rmp : Gain  Gain=60/(2*pi)
  "Propeller model " : MATLAB Function  TreatAsAtomicUnit=on  SystemSampleTime=octomodel.sampletime
  torque : Outport  VectorParamsAs1DForOutWhenUnconnected=off
  thrusth : Outport  Port=2  VectorParamsAs1DForOutWhenUnconnected=off
  wires:
  "Propeller model "/1(torque) -> torque/1
  "Propeller model "/2(thrust) -> thrusth/1
  w angular speed/1 -> Convert rad/s to rmp/1
  Convert rad/s to rmp/1 -> "Propeller model "/1(rpm)

== system complete/Motors/DC Motor 6/Mechanical part/speed - torque load relationship we will not consider for now ==
  w angular speed : Inport
  Convert rad/s to rmp : Gain  Gain=60/(2*pi)
  "Propeller model " : MATLAB Function  TreatAsAtomicUnit=on  SystemSampleTime=octomodel.sampletime
  torque : Outport  VectorParamsAs1DForOutWhenUnconnected=off
  thrusth : Outport  Port=2  VectorParamsAs1DForOutWhenUnconnected=off
  wires:
  Convert rad/s to rmp/1 -> "Propeller model "/1(rpm)
  w angular speed/1 -> Convert rad/s to rmp/1
  "Propeller model "/2(thrust) -> thrusth/1
  "Propeller model "/1(torque) -> torque/1

== system complete/Motors/DC Motor 7/Mechanical part/speed - torque load relationship we will not consider for now ==
  w angular speed : Inport
  Convert rad/s to rmp : Gain  Gain=60/(2*pi)
  "Propeller model " : MATLAB Function  TreatAsAtomicUnit=on  SystemSampleTime=octomodel.sampletime
  torque : Outport  VectorParamsAs1DForOutWhenUnconnected=off
  thrusth : Outport  Port=2  VectorParamsAs1DForOutWhenUnconnected=off
  wires:
  "Propeller model "/1(torque) -> torque/1
  "Propeller model "/2(thrust) -> thrusth/1
  w angular speed/1 -> Convert rad/s to rmp/1
  Convert rad/s to rmp/1 -> "Propeller model "/1(rpm)

== matlab function complete/Motors/DC Motor 1/Mechanical part/speed - torque load relationship we will not consider for now/Propeller model  ==
  data: torque output; rpm input; thrust output
function [torque,thrust] = fcn(rpm)
% angular_velocity in rpm
if rpm>2000
    see=1;
end
%coefficient of thrust, empirically derived
coef_t = 0.0524;
%thrust = coef_t * density of air * velocity^2 * propeller diameter (m) ^4
%velocity in rev/sec, where  1 rev/sec = 1 rpm/60
thrust = coef_t*1.225*(rpm/60)^2*.381^4; % 15 inches ~ 0.381 m
% empirically derived
torque = (1.065e-08)*rpm^2 + (-3.45e-06)*rpm + (0.0064);

end
